simulink model "model_2"  (R2020a)
settings: Solver=VariableStepAuto  StartTime=0.0  StopTime=10.0  RelTol=1e-3
settings Model: Creator=Notnik_kg  LastModifiedBy=Notnik_kg

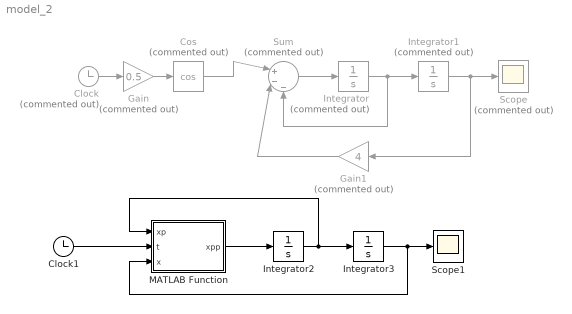
== system model_2 ==
  Clock : Clock  Commented=on
  Clock1 : Clock
  Cos : Trigonometry  Commented=on  Operator=cos
  Gain : Gain  Commented=on  Gain=0.5
  Gain1 : Gain  Commented=on  Gain=4
  Integrator : Integrator  Commented=on  InitialCondition=1
  Integrator1 : Integrator  Commented=on  InitialCondition=1
  Integrator2 : Integrator  InitialCondition=1
  Integrator3 : Integrator  InitialCondition=1
  MATLAB Function : MATLAB Function  TreatAsAtomicUnit=on
  Scope : Scope  Commented=on
  Scope1 : Scope
  Sum : Sum  Commented=on  Inputs=|+--
  wires:
  Clock/1 -> Gain/1
  Gain/1 -> Cos/1
  Cos/1 -> Sum/1
  Sum/1 -> Integrator/1
  Integrator/1 -> Sum/3, Integrator1/1
  Integrator1/1 -> Gain1/1, Scope/1
  Gain1/1 -> Sum/2
  Clock1/1 -> MATLAB Function/2(t)
  MATLAB Function/1(xpp) -> Integrator2/1
  Integrator2/1 -> MATLAB Function/1(xp), Integrator3/1
  Integrator3/1 -> Scope1/1, MATLAB Function/3(x)

== matlab function model_2/MATLAB Function ==
  data: xp input; t input; x input; xpp output
function xpp = fcn(xp, t, x)
xpp = cos(0.5.*t) - xp - 4.*x;
